simulink model "Spange_Thrust_simulation"  (R2016a)
settings: Solver=ode3  StartTime=0.0  StopTime=4  RelTol=1e-3
values from neighbouring files (symbols this model uses):
  C = [C1;C2;C3]    [Spange_init.m]
  D = 3.0/100    (= 0.03)    [Spange_init.m]
  eps_c = 5    [Spange_init.m]
  epsilon = 0.5    [Spange_init.m]
  hd = c2d(H1,0.1,'foh')    [Spange_init.m]
  hd2 = c2d(H2,0.01,'zoh')    [Spange_init.m]
  I_s = 0.05    [Spange_init.m]
  k_cc = 1    [Spange_init.m]
  K_omega = 0.3    [Spange_init.m]
  K_q1f = 0.0113    [Spange_init.m]
  K_q1r = K_q1f    (= 0.0113)    [Spange_init.m]
  K_q2f = 0.0117    [Spange_init.m]
  K_q2r = K_q2f    (= 0.0117)    [Spange_init.m]
  K_q3f = 0.0113    [Spange_init.m]
  K_q3r = K_q3f    (= 0.0113)    [Spange_init.m]
  K_T1f = 0.3763    [Spange_init.m]
  K_T1r = K_T1f    (= 0.3763)    [Spange_init.m]
  K_T2f = 0.3901    [Spange_init.m]
  K_T2r = K_T2f    (= 0.3901)    [Spange_init.m]
  K_T3f = 0.3776    [Spange_init.m]
  K_T3r = K_T3f    (= 0.3776)    [Spange_init.m]
  Kp = 0.3    [Spange_init.m]
  Max_Acceleration = 2    [Spange_init.m]
  Max_rotation = 12*sqrt(lambda)    [Spange_init.m]
  Max_thrust = 1.5034    [Spange_init.m]
  Min_thrust = -0.85    [Spange_init.m]
  n_c = 5    [Spange_init.m]
  n_max = 64.6    [Spange_init.m]
  p_cc = 0.5    [Spange_init.m]
  Q_f0 = 0.3    [Spange_init.m]
  r_cc = 4    [Spange_init.m]
  Rho = Rho_m    (= 1000)    [Spange_init.m]
  tc = [u(1),u(2),u(3)]'    [Spange_thrustallocationQuadratic_mode1.m]    (also in Spange_thrustallocationQuadratic_mode2.m; Spange_thrustallocationQuadratic_mode3.m; Spange_thrustallocationQuadratic_mode4.m)
  Thruster_control = 1    [Spange_init.m]
  u_e = [1 0 1 0 0 ... (first row only)    [Spange_init.m]
undefined symbols (not defined in the file or in its folder): Thruster
libraries: simulink_extras x4, simulink x3
settings Model: Creator=Joachim  LastModifiedBy=Joachim
settings DataIOCC: LimitDataPoints=on

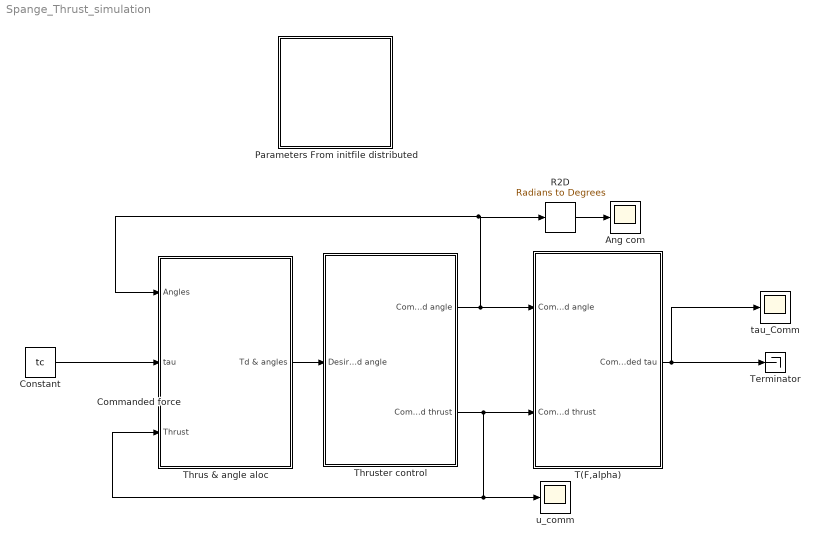
== system Spange_Thrust_simulation ==
  Ang com : Scope
  Commanded force : Constant  Value=tc
  Constant : Constant  Value=tc
  "Parameters From initfile distributed " : Subsystem
  R2D : simulink_extras/Transformations/Radians to Degrees
  T(F,alpha) : Subsystem
  Terminator : Terminator
  Thrus & angle aloc : Subsystem
  Thruster control : Subsystem
  tau_Comm : Scope
  u_comm : Scope
  wires:
  Thrus & angle aloc/1(Td & angles) -> Thruster control/1("Desired thrust and angle ")
  T(F,alpha)/1(Commanded tau) -> Terminator/1, tau_Comm/1
  R2D/1 -> Ang com/1
  Thruster control/2("Commanded thrust ") -> u_comm/1, Thrus & angle aloc/3(Thrust), T(F,alpha)/2(Commanded thrust)
  Thruster control/1(Commanded angle) -> T(F,alpha)/1(Commanded angle), R2D/1, Thrus & angle aloc/1(Angles)
  Constant/1 -> Thrus & angle aloc/2(tau)

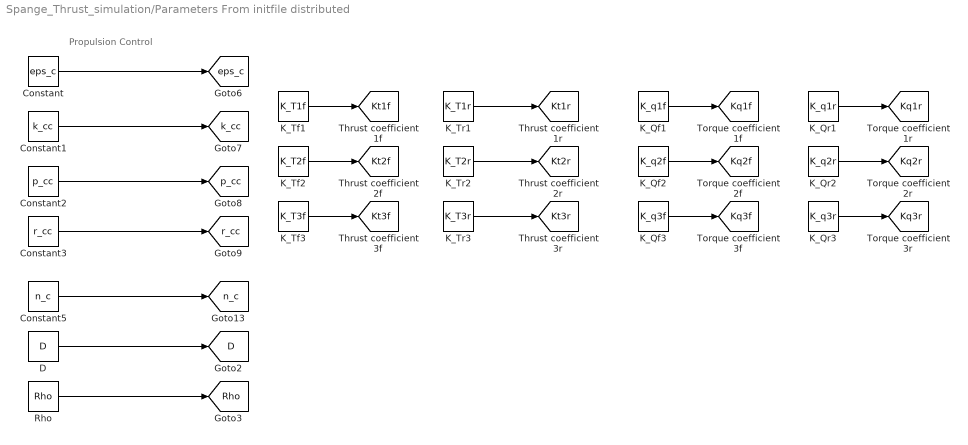
== system Spange_Thrust_simulation/Parameters From initfile distributed  ==
  note: Propulsion Control
  Constant : Constant  Value=eps_c
  Constant1 : Constant  Value=k_cc
  Constant2 : Constant  Value=p_cc
  Constant3 : Constant  Value=r_cc
  Constant5 : Constant  Value=n_c
  D : Constant  Value=D
  K_Qf1 : Constant  Value=K_q1f
  K_Qf2 : Constant  Value=K_q2f
  K_Qf3 : Constant  Value=K_q3f
  K_Qr1 : Constant  Value=K_q1r
  K_Qr2 : Constant  Value=K_q2r
  K_Qr3 : Constant  Value=K_q3r
  K_Tf1 : Constant  Value=K_T1f
  K_Tf2 : Constant  Value=K_T2f
  K_Tf3 : Constant  Value=K_T3f
  K_Tr1 : Constant  Value=K_T1r
  K_Tr2 : Constant  Value=K_T2r
  K_Tr3 : Constant  Value=K_T3r
  Rho : Constant  Value=Rho
  tag scope: D=global, Kq1f=global, Kq1r=global, Kq2f=global, Kq2r=global, Kq3f=global, Kq3r=global, Kt1f=global, Kt1r=global, Kt2f=global, Kt2r=global, Kt3f=global, Kt3r=global, Rho=global, eps_c=global, k_cc=global, n_c=global, p_cc=global, r_cc=global
  wires:
  D/1 -> [D]
  Rho/1 -> [Rho]
  Constant/1 -> [eps_c]
  Constant1/1 -> [k_cc]
  Constant2/1 -> [p_cc]
  Constant3/1 -> [r_cc]
  Constant5/1 -> [n_c]
  K_Tf1/1 -> [Kt1f]
  K_Tf3/1 -> [Kt3f]
  K_Tf2/1 -> [Kt2f]
  K_Tr1/1 -> [Kt1r]
  K_Tr2/1 -> [Kt2r]
  K_Tr3/1 -> [Kt3r]
  K_Qf1/1 -> [Kq1f]
  K_Qf2/1 -> [Kq2f]
  K_Qf3/1 -> [Kq3f]
  K_Qr1/1 -> [Kq1r]
  K_Qr2/1 -> [Kq2r]
  K_Qr3/1 -> [Kq3r]

== system Spange_Thrust_simulation/T(F,alpha) ==
  Commanded angle : Inport
  Commanded thrust : Inport  Port=2
  MATLAB Function : MATLAB Function  TreatAsAtomicUnit=on
  Radians to Degrees : simulink_extras/Transformations/Radians to Degrees
  X-position Thruster : Constant  Value=[Thruster.T1(1) Thruster.T2(1) Thruster.T3(1)]
  Y-position Thruster : Constant  Value=[Thruster.T1(2) Thruster.T2(2) Thruster.T3(2)]
  Commanded tau : Outport
  wires:
  Commanded angle/1 -> Radians to Degrees/1
  X-position Thruster/1 -> MATLAB Function/3(PosX)
  Y-position Thruster/1 -> MATLAB Function/4(PosY)
  MATLAB Function/1(actual_tau) -> Commanded tau/1
  Commanded thrust/1 -> MATLAB Function/1(thrust_actual)
  Radians to Degrees/1 -> MATLAB Function/2(alpha_actual)

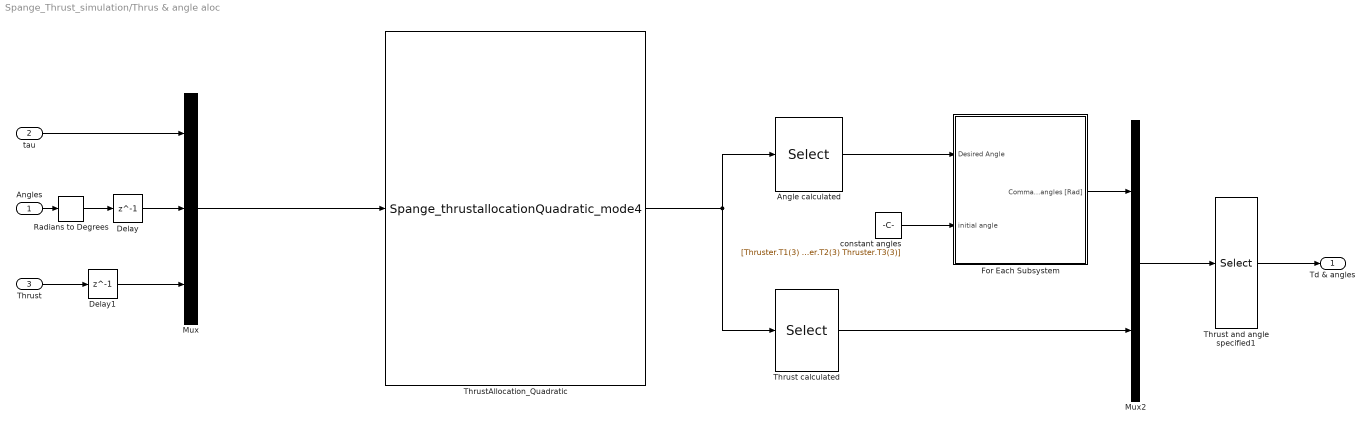
== system Spange_Thrust_simulation/Thrus & angle aloc ==
  Angles : Inport
  tau : Inport  Port=2
  Thrust : Inport  Port=3
  "  Thrust calculated" : Selector  InputPortWidth=6  IndexOptions=Index vector (dialog)  Indices=[4 5 6]  OutputSizes=1
  " Angle calculated" : Selector  InputPortWidth=6  IndexOptions=Index vector (dialog)  Indices=[1 2 3]  OutputSizes=1
  Delay : Delay  DelayLength=1  InitialCondition=[Thruster.T1(3) Thruster.T2(3) Thruster.T3(3)]
  Delay1 : Delay  DelayLength=1  InitialCondition=[0,0,0]
  For Each Subsystem : Subsystem  TreatAsAtomicUnit=on
  Mux : Mux  Inputs=3
  Mux2 : Mux  Inputs=2
  Radians to Degrees : simulink_extras/Transformations/Radians to Degrees
  Thrust and angle specified1 : Selector  InputPortWidth=6  IndexOptions=Index vector (dialog)  Indices=[4 1 5 2 6 3]  OutputSizes=1
  ThrustAllocation_Quadratic : S-Function  RequirementInfo={} %GIDa_b9c7dd03_57d1_40a3_b341_131bae047cf5  FunctionName=Spange_thrustallocationQuadratic_mode4  Parameters=u_e,Thruster,C  SFunctionDeploymentMode=off  EnableBusSupport=off
  constant angles : Constant  Value=[Thruster.T1(3) Thruster.T2(3) Thruster.T3(3)]
  Td & angles : Outport
  wires:
  tau/1 -> Mux/1
  Angles/1 -> Radians to Degrees/1
  Radians to Degrees/1 -> Delay/1
  Thrust/1 -> Delay1/1
  Delay/1 -> Mux/2
  Thrust and angle specified1/1 -> Td & angles/1
  Mux2/1 -> Thrust and angle specified1/1
  " Angle calculated"/1 -> For Each Subsystem/1(Desired Angle)
  For Each Subsystem/1("Commanded angles [Rad] ") -> Mux2/1
  constant angles/1 -> For Each Subsystem/2("initial angle ")
  "  Thrust calculated"/1 -> Mux2/2
  ThrustAllocation_Quadratic/1 -> " Angle calculated"/1, "  Thrust calculated"/1
  Delay1/1 -> Mux/3
  Mux/1 -> ThrustAllocation_Quadratic/1

== system Spange_Thrust_simulation/Thruster control ==
  "Desired thrust and angle " : Inport
  Demux : Demux  Outputs=6
  Mux : Mux  Inputs=6
  Selecting Actual thrust : Selector  InputPortWidth=6  IndexOptions=Index vector (dialog)  Indices=[1 3 5]  OutputSizes=1
  Selecting actual angle : Selector  InputPortWidth=6  IndexOptions=Index vector (dialog)  Indices=[2 4 6]  OutputSizes=1
  Subsystem : Subsystem
  Thruster 1 : Subsystem
      settings: AttributesFormatString=%<MinAlgLoopOccurrences>
  Thruster 2 : Subsystem
      settings: AttributesFormatString=%<MinAlgLoopOccurrences>
  Thruster 3 : Subsystem
      settings: AttributesFormatString=%<MinAlgLoopOccurrences>
  Commanded angle : Outport
  "Commanded thrust " : Outport  Port=2
  wires:
  Demux/1 -> Thruster 1/1(Desired thrust 1)
  Selecting Actual thrust/1 -> Subsystem/1(Calculated thrust)
  Subsystem/1(Thrust from model) -> "Commanded thrust "/1
  Selecting actual angle/1 -> Commanded angle/1
  Thruster 1/2(Commanded angle) -> Mux/2
  Demux/2 -> Thruster 1/2(Desired Angle)
  Mux/1 -> Selecting Actual thrust/1, Selecting actual angle/1
  Thruster 3/2(Commanded angle) -> Mux/6
  Thruster 3/1("Commanded thrust ") -> Mux/5
  Thruster 2/2(Commanded angle) -> Mux/4
  Thruster 2/1(Commanded thrust 1) -> Mux/3
  Thruster 1/1(Commanded thrust 1) -> Mux/1
  Demux/6 -> Thruster 3/2(Desired Angle)
  Demux/5 -> Thruster 3/1(Desired thrust 1)
  Demux/4 -> Thruster 2/2(Desired Angle)
  Demux/3 -> Thruster 2/1(Desired thrust 1)
  "Desired thrust and angle "/1 -> Demux/1

== system Spange_Thrust_simulation/Thrus & angle aloc/For Each Subsystem ==
  Desired Angle : Inport  Partition=on  PartitionDimension=1  PartitionWidth=1
  "initial angle " : Inport  Port=2  Partition=on  PartitionDimension=1  PartitionWidth=1
  Degrees to Radians : simulink_extras/Transformations/Degrees to Radians
  Ensures fastest way is chosen : MATLAB Function  TreatAsAtomicUnit=on
  For Each : ForEach  DisableCoverage=on  IndexMode=One-based
  Integrator : Integrator  ExternalReset=either  InitialConditionSource=external
  MATLAB Function : MATLAB Function  TreatAsAtomicUnit=on
  Max Rotation Rate : Saturate  UpperLimit=Max_rotation  LowerLimit=-Max_rotation
  constant : Constant  Value=0
  "Commanded angles [Rad] " : Outport  ConcatenationDimension=1
  wires:
  Degrees to Radians/1 -> MATLAB Function/1(angle)
  MATLAB Function/1(y) -> "Commanded angles [Rad] "/1
  Integrator/1 -> Degrees to Radians/1, Ensures fastest way is chosen/2(actual)  "angle"
  "initial angle "/1 -> Integrator/3
  Max Rotation Rate/1 -> Integrator/1
  Ensures fastest way is chosen/1(psi_D) -> Max Rotation Rate/1
  Desired Angle/1 -> Ensures fastest way is chosen/1(desired)
  constant/1 -> Integrator/2

== system Spange_Thrust_simulation/Thruster control/Subsystem ==
  Calculated thrust : Inport
  Demux : Demux  Outputs=3
  Mux : Mux  Inputs=3
  Saturation 1 : Saturate  UpperLimit=Max_thrust  LowerLimit=Min_thrust
  Saturation 2 : Saturate  UpperLimit=Max_thrust  LowerLimit=Min_thrust
  Saturation 3 : Saturate  UpperLimit=Max_thrust  LowerLimit=Min_thrust
  Thrust from model : Outport
  wires:
  Saturation 2/1 -> Mux/2
  Saturation 3/1 -> Mux/3
  Saturation 1/1 -> Mux/1
  Mux/1 -> Thrust from model/1
  Demux/3 -> Saturation 3/1
  Demux/2 -> Saturation 2/1
  Demux/1 -> Saturation 1/1
  Calculated thrust/1 -> Demux/1

== system Spange_Thrust_simulation/Thruster control/Thruster 1 ==
  Desired thrust 1 : Inport
  Desired Angle : Inport  Port=2
  Constant : Constant  Value=hd2.den{1,1}
  Constant1 : Constant  Value=hd2.num{1,1}
  Discrete Transfer Fcn : DiscreteTransferFcn  NumeratorSource=Input port  DenominatorSource=Input port  Denominator=[0.2 1]  SampleTime=0.01  a0EqualsOne=on
      settings: InputPortMap=u0,p1,p3
  Losses (placeholder) : Constant  Value=0
  Propeller Hydrodynamics : Subsystem
  Shaft dynamics : Subsystem
  Thruster control : Subsystem
  Commanded thrust 1 : Outport
  Commanded angle : Outport  Port=2
  wires:
  Desired thrust 1/1 -> Thruster control/1("T_d ")
  Discrete Transfer Fcn/1 -> Shaft dynamics/1(Qm)
  Propeller Hydrodynamics/2(Qa) -> Shaft dynamics/2(Qa)
  Shaft dynamics/1(n) -> Propeller Hydrodynamics/2(n), Thruster control/2(n)
  Constant/1 -> Discrete Transfer Fcn/3
  Constant1/1 -> Discrete Transfer Fcn/2
  Desired Angle/1 -> Commanded angle/1
  Thruster control/1(Qc) -> Discrete Transfer Fcn/1
  Propeller Hydrodynamics/1(Ta) -> Commanded thrust 1/1
  Losses (placeholder)/1 -> Propeller Hydrodynamics/1(env)

== system Spange_Thrust_simulation/Thruster control/Thruster 2 ==
  Desired thrust 1 : Inport
  Desired Angle : Inport  Port=2
  Constant : Constant  Value=hd2.den{1,1}
  Constant1 : Constant  Value=hd2.num{1,1}
  Discrete Transfer Fcn : DiscreteTransferFcn  NumeratorSource=Input port  DenominatorSource=Input port  Denominator=[0.2 1]  SampleTime=0.01  a0EqualsOne=on
      settings: InputPortMap=u0,p1,p3
  Losses (placeholder) : Constant  Value=0
  Propeller Hydrodynamics : Subsystem
  Shaft dynamics : Subsystem
  Thruster control : Subsystem
  Commanded thrust 1 : Outport
  Commanded angle : Outport  Port=2
  wires:
  Propeller Hydrodynamics/2(Qa) -> Shaft dynamics/2(Qa)
  Shaft dynamics/1(n) -> Propeller Hydrodynamics/2(n), Thruster control/2(n)
  Constant/1 -> Discrete Transfer Fcn/3
  Constant1/1 -> Discrete Transfer Fcn/2
  Desired Angle/1 -> Commanded angle/1
  Propeller Hydrodynamics/1(Ta) -> Commanded thrust 1/1
  Desired thrust 1/1 -> Thruster control/1("T_d ")
  Discrete Transfer Fcn/1 -> Shaft dynamics/1(Qm)
  Thruster control/1(Qc) -> Discrete Transfer Fcn/1
  Losses (placeholder)/1 -> Propeller Hydrodynamics/1(env)

== system Spange_Thrust_simulation/Thruster control/Thruster 3 ==
  Desired thrust 1 : Inport
  Desired Angle : Inport  Port=2
  Constant : Constant  Value=hd2.den{1,1}
  Constant1 : Constant  Value=hd2.num{1,1}
  Discrete Transfer Fcn : DiscreteTransferFcn  NumeratorSource=Input port  DenominatorSource=Input port  Denominator=[0.2 1]  SampleTime=0.01  a0EqualsOne=on
      settings: InputPortMap=u0,p1,p3
  Losses (placeholder) : Constant  Value=0
  Propeller Hydrodynamics : Subsystem
  Shaft dynamics : Subsystem
  Thruster control : Subsystem
  "Commanded thrust " : Outport
  Commanded angle : Outport  Port=2
  wires:
  Propeller Hydrodynamics/2(Qa) -> Shaft dynamics/2(Qa)
  Shaft dynamics/1(n) -> Propeller Hydrodynamics/2(n), Thruster control/2(n)
  Constant/1 -> Discrete Transfer Fcn/3
  Constant1/1 -> Discrete Transfer Fcn/2
  Desired Angle/1 -> Commanded angle/1
  Propeller Hydrodynamics/1(Ta) -> "Commanded thrust "/1
  Desired thrust 1/1 -> Thruster control/1("T_d ")
  Discrete Transfer Fcn/1 -> Shaft dynamics/1(Qm)
  Thruster control/1(Qc) -> Discrete Transfer Fcn/1
  Losses (placeholder)/1 -> Propeller Hydrodynamics/1(env)

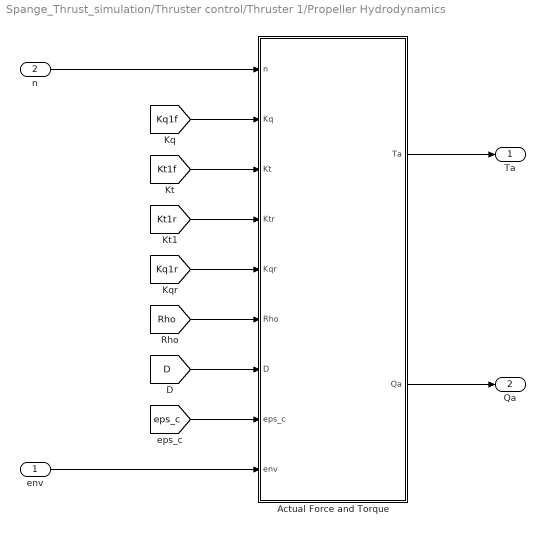
== system Spange_Thrust_simulation/Thruster control/Thruster 1/Propeller Hydrodynamics ==
  env : Inport
  n : Inport  Port=2
  Actual Force and Torque : MATLAB Function  TreatAsAtomicUnit=on
  Ta : Outport
  Qa : Outport  Port=2
  wires:
  [eps_c] -> Actual Force and Torque/8(eps_c)
  [Kq1r] -> Actual Force and Torque/5(Kqr)
  [Kt1r] -> Actual Force and Torque/4(Ktr)
  Actual Force and Torque/1(Ta) -> Ta/1
  [Kt1f] -> Actual Force and Torque/3(Kt)
  env/1 -> Actual Force and Torque/9(env)
  [Rho] -> Actual Force and Torque/6(Rho)
  Actual Force and Torque/2(Qa) -> Qa/1
  [Kq1f] -> Actual Force and Torque/2(Kq)
  [D] -> Actual Force and Torque/7(D)
  n/1 -> Actual Force and Torque/1(n)

== system Spange_Thrust_simulation/Thruster control/Thruster 1/Shaft dynamics ==
  Qm : Inport
  Qa : Inport  Port=2
  Constant : Constant  Value=0
  Finding rotation speed : Gain  Gain=1/(2*pi*I_s)
  Integrator : Integrator  ExternalReset=either
  K_omega : Gain  Gain=K_omega*2*pi
  Sum : Sum  Inputs=-+-
  n : Outport
  wires:
  Constant/1 -> Integrator/2
  Integrator/1 -> K_omega/1, n/1
  Finding rotation speed/1 -> Integrator/1
  K_omega/1 -> Sum/3
  Qa/1 -> Sum/1
  Sum/1 -> Finding rotation speed/1
  Qm/1 -> Sum/2

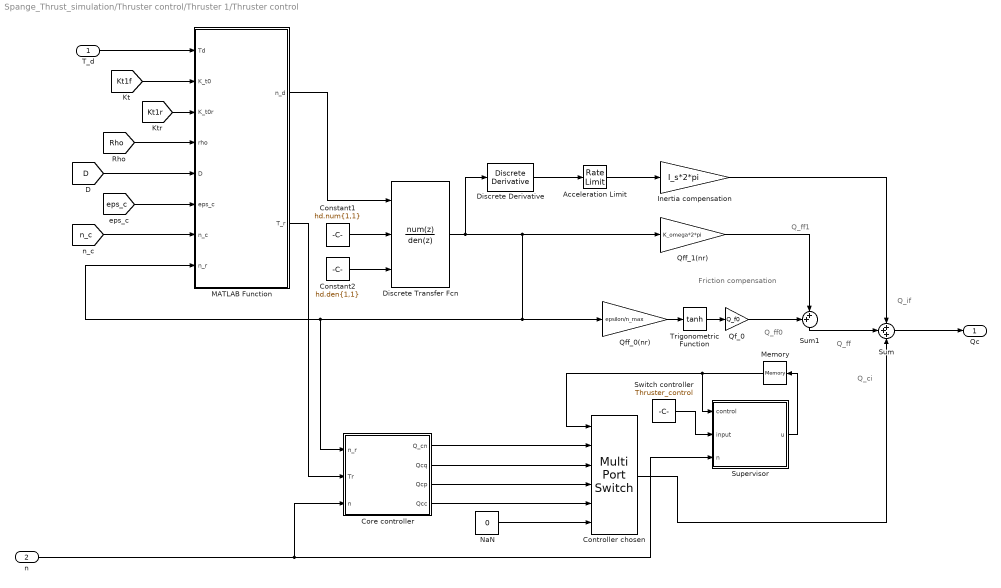
== system Spange_Thrust_simulation/Thruster control/Thruster 1/Thruster control ==
  note: Friction compensation
  note: Q_ff1
  note: Q_ff0
  note: Q_ff
  note: Q_if
  note: Q_ci
  "T_d " : Inport
  n : Inport  Port=2
  Acceleration Limit : RateLimiter  RisingSlewLimit=Max_Acceleration  FallingSlewLimit=-Max_Acceleration  SampleTimeMode=inherited
  Constant1 : Constant  Value=hd.num{1,1}  VectorParams1D=off
  Constant2 : Constant  Value=hd.den{1,1}  VectorParams1D=off
  Controller chosen : MultiPortSwitch  Inputs=5
  Core controller : Subsystem
  Discrete Transfer Fcn : DiscreteTransferFcn  NumeratorSource=Input port  Numerator=[8.76e-05 0.0003481 8.648e-05]  DenominatorSource=Input port  Denominator=[1 -1.974 0.9746]  SampleTime=0.01  a0EqualsOne=on
      settings: InputPortMap=u0,p1,p3
  Discrete Derivative : simulink/Discrete/Discrete Derivative  gainval=1.0  ICPrevScaledInput=0.0  InputProcessing=Inherited  OutMin=[]  OutMax=[]  OutDataType=fixdt(1, 16)  OutScaling=2^-10  DoSatur=off
  Inertia compensation : Gain  Gain=I_s*2*pi
  MATLAB Function : MATLAB Function  TreatAsAtomicUnit=on
  Memory : Memory  X0=1  InheritSampleTime=on
  NaN : Constant  Value=0
  Qf_0 : Gain  Gain=Q_f0
  Qff_0(nr) : Gain  Gain=epsilon/n_max
  Qff_1(nr) : Gain  Gain=K_omega*2*pi
  Sum : Sum  Inputs=+++
  Sum1 : Sum  Inputs=++|
  Supervisor : MATLAB Function  TreatAsAtomicUnit=on
  Switch controller : Constant  Value=Thruster_control
  Trigonometric Function : Trigonometry  Operator=tanh
  Qc : Outport
  wires:
  Sum/1 -> Qc/1
  [Kt1r] -> MATLAB Function/3(K_t0r)
  [Kt1f] -> MATLAB Function/2(K_t0)
  "T_d "/1 -> MATLAB Function/1(Td)
  Discrete Transfer Fcn/1 -> Discrete Derivative/1, Qff_1(nr)/1, Qff_0(nr)/1, MATLAB Function/8(n_r), Core controller/1(n_r)
  Acceleration Limit/1 -> Inertia compensation/1
  n/1 -> Supervisor/3(n), Core controller/3("n ")
  Inertia compensation/1 -> Sum/1
  Constant2/1 -> Discrete Transfer Fcn/3
  Constant1/1 -> Discrete Transfer Fcn/2
  Sum1/1 -> Sum/2
  Discrete Derivative/1 -> Acceleration Limit/1
  [n_c] -> MATLAB Function/7(n_c)
  Core controller/1(Q_cn) -> Controller chosen/2
  Core controller/4(Qcc) -> Controller chosen/5
  Core controller/3(Qcp) -> Controller chosen/4
  Core controller/2(Qcq) -> Controller chosen/3
  Controller chosen/1 -> Sum/3
  Switch controller/1 -> Supervisor/2(input)
  Qf_0/1 -> Sum1/1
  Qff_1(nr)/1 -> Sum1/2
  Memory/1 -> Supervisor/1(control), Controller chosen/1
  Supervisor/1(u) -> Memory/1
  NaN/1 -> Controller chosen/6
  Trigonometric Function/1 -> Qf_0/1
  Qff_0(nr)/1 -> Trigonometric Function/1
  MATLAB Function/1(n_d) -> Discrete Transfer Fcn/1
  MATLAB Function/2(T_r) -> Core controller/2("Tr ")
  [eps_c] -> MATLAB Function/6(eps_c)
  [D] -> MATLAB Function/5(D)
  [Rho] -> MATLAB Function/4(rho)

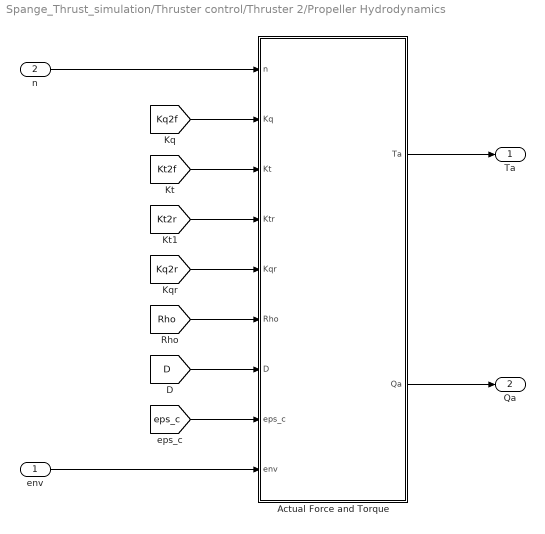
== system Spange_Thrust_simulation/Thruster control/Thruster 2/Propeller Hydrodynamics ==
  env : Inport
  n : Inport  Port=2
  Actual Force and Torque : MATLAB Function  TreatAsAtomicUnit=on
  Ta : Outport
  Qa : Outport  Port=2
  wires:
  [eps_c] -> Actual Force and Torque/8(eps_c)
  [Kq2r] -> Actual Force and Torque/5(Kqr)
  [Kt2r] -> Actual Force and Torque/4(Ktr)
  Actual Force and Torque/1(Ta) -> Ta/1
  [Kt2f] -> Actual Force and Torque/3(Kt)
  env/1 -> Actual Force and Torque/9(env)
  [Rho] -> Actual Force and Torque/6(Rho)
  Actual Force and Torque/2(Qa) -> Qa/1
  [Kq2f] -> Actual Force and Torque/2(Kq)
  [D] -> Actual Force and Torque/7(D)
  n/1 -> Actual Force and Torque/1(n)

== system Spange_Thrust_simulation/Thruster control/Thruster 2/Shaft dynamics ==
  Qm : Inport
  Qa : Inport  Port=2
  Constant : Constant  Value=0
  Finding rotation speed : Gain  Gain=1/(2*pi*I_s)
  Integrator : Integrator  ExternalReset=either
  K_omega : Gain  Gain=K_omega*2*pi
  Sum : Sum  Inputs=-+-
  n : Outport
  wires:
  Constant/1 -> Integrator/2
  Integrator/1 -> n/1, K_omega/1
  Finding rotation speed/1 -> Integrator/1
  K_omega/1 -> Sum/3
  Qa/1 -> Sum/1
  Sum/1 -> Finding rotation speed/1
  Qm/1 -> Sum/2

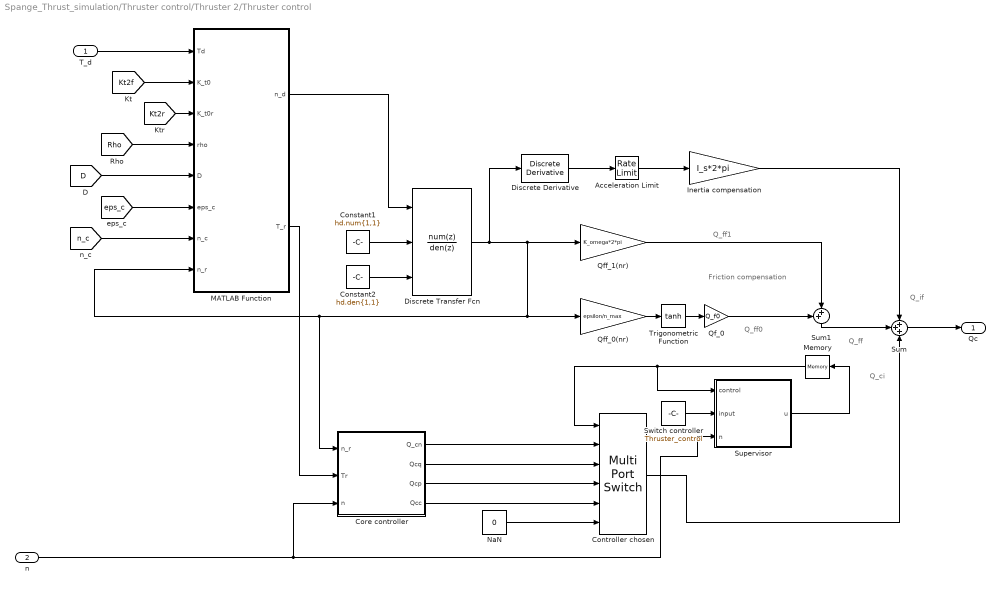
== system Spange_Thrust_simulation/Thruster control/Thruster 2/Thruster control ==
  note: Friction compensation
  note: Q_ff1
  note: Q_ff0
  note: Q_ff
  note: Q_if
  note: Q_ci
  "T_d " : Inport
  n : Inport  Port=2
  Acceleration Limit : RateLimiter  RisingSlewLimit=Max_Acceleration  FallingSlewLimit=-Max_Acceleration  SampleTimeMode=inherited
  Constant1 : Constant  Value=hd.num{1,1}  VectorParams1D=off
  Constant2 : Constant  Value=hd.den{1,1}  VectorParams1D=off
  Controller chosen : MultiPortSwitch  Inputs=5
  Core controller : Subsystem
  Discrete Transfer Fcn : DiscreteTransferFcn  NumeratorSource=Input port  Numerator=[8.76e-05 0.0003481 8.648e-05]  DenominatorSource=Input port  Denominator=[1 -1.974 0.9746]  SampleTime=0.01  a0EqualsOne=on
      settings: InputPortMap=u0,p1,p3
  Discrete Derivative : simulink/Discrete/Discrete Derivative  gainval=1.0  ICPrevScaledInput=0.0  InputProcessing=Inherited  OutMin=[]  OutMax=[]  OutDataType=fixdt(1, 16)  OutScaling=2^-10  DoSatur=off
  Inertia compensation : Gain  Gain=I_s*2*pi
  MATLAB Function : MATLAB Function  TreatAsAtomicUnit=on
  Memory : Memory  X0=1
  NaN : Constant  Value=0
  Qf_0 : Gain  Gain=Q_f0
  Qff_0(nr) : Gain  Gain=epsilon/n_max
  Qff_1(nr) : Gain  Gain=K_omega*2*pi
  Sum : Sum  Inputs=+++
  Sum1 : Sum  Inputs=++|
  Supervisor : MATLAB Function  TreatAsAtomicUnit=on
  Switch controller : Constant  Value=Thruster_control
  Trigonometric Function : Trigonometry  Operator=tanh
  Qc : Outport
  wires:
  [Kt2r] -> MATLAB Function/3(K_t0r)
  [Kt2f] -> MATLAB Function/2(K_t0)
  Sum/1 -> Qc/1
  Discrete Transfer Fcn/1 -> Qff_1(nr)/1, Core controller/1(n_r), MATLAB Function/8(n_r), Qff_0(nr)/1, Discrete Derivative/1
  Acceleration Limit/1 -> Inertia compensation/1
  n/1 -> Supervisor/3(n), Core controller/3("n ")
  Discrete Derivative/1 -> Acceleration Limit/1
  MATLAB Function/1(n_d) -> Discrete Transfer Fcn/1
  Constant2/1 -> Discrete Transfer Fcn/3
  Constant1/1 -> Discrete Transfer Fcn/2
  [n_c] -> MATLAB Function/7(n_c)
  [eps_c] -> MATLAB Function/6(eps_c)
  [D] -> MATLAB Function/5(D)
  [Rho] -> MATLAB Function/4(rho)
  "T_d "/1 -> MATLAB Function/1(Td)
  Switch controller/1 -> Supervisor/2(input)
  Core controller/2(Qcq) -> Controller chosen/3
  Core controller/3(Qcp) -> Controller chosen/4
  Inertia compensation/1 -> Sum/1
  Controller chosen/1 -> Sum/3
  Qf_0/1 -> Sum1/1
  Qff_1(nr)/1 -> Sum1/2
  Memory/1 -> Controller chosen/1, Supervisor/1(control)
  Supervisor/1(u) -> Memory/1
  NaN/1 -> Controller chosen/6
  Core controller/4(Qcc) -> Controller chosen/5
  Core controller/1(Q_cn) -> Controller chosen/2
  Sum1/1 -> Sum/2
  Trigonometric Function/1 -> Qf_0/1
  Qff_0(nr)/1 -> Trigonometric Function/1
  MATLAB Function/2(T_r) -> Core controller/2("Tr ")

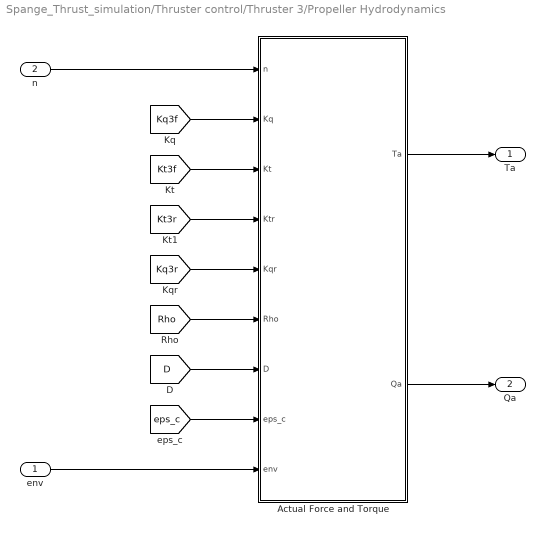
== system Spange_Thrust_simulation/Thruster control/Thruster 3/Propeller Hydrodynamics ==
  env : Inport
  n : Inport  Port=2
  Actual Force and Torque : MATLAB Function  TreatAsAtomicUnit=on
  Ta : Outport
  Qa : Outport  Port=2
  wires:
  [eps_c] -> Actual Force and Torque/8(eps_c)
  [Kq3r] -> Actual Force and Torque/5(Kqr)
  [Kt3r] -> Actual Force and Torque/4(Ktr)
  Actual Force and Torque/1(Ta) -> Ta/1
  [Kt3f] -> Actual Force and Torque/3(Kt)
  env/1 -> Actual Force and Torque/9(env)
  [Rho] -> Actual Force and Torque/6(Rho)
  Actual Force and Torque/2(Qa) -> Qa/1
  [Kq3f] -> Actual Force and Torque/2(Kq)
  [D] -> Actual Force and Torque/7(D)
  n/1 -> Actual Force and Torque/1(n)

== system Spange_Thrust_simulation/Thruster control/Thruster 3/Shaft dynamics ==
  Qm : Inport
  Qa : Inport  Port=2
  Constant : Constant  Value=0
  Finding rotation speed : Gain  Gain=1/(2*pi*I_s)
  Integrator : Integrator  ExternalReset=either
  K_omega : Gain  Gain=K_omega*2*pi
  Sum : Sum  Inputs=-+-
  n : Outport
  wires:
  Constant/1 -> Integrator/2
  Integrator/1 -> K_omega/1, n/1
  Finding rotation speed/1 -> Integrator/1
  K_omega/1 -> Sum/3
  Qa/1 -> Sum/1
  Sum/1 -> Finding rotation speed/1
  Qm/1 -> Sum/2

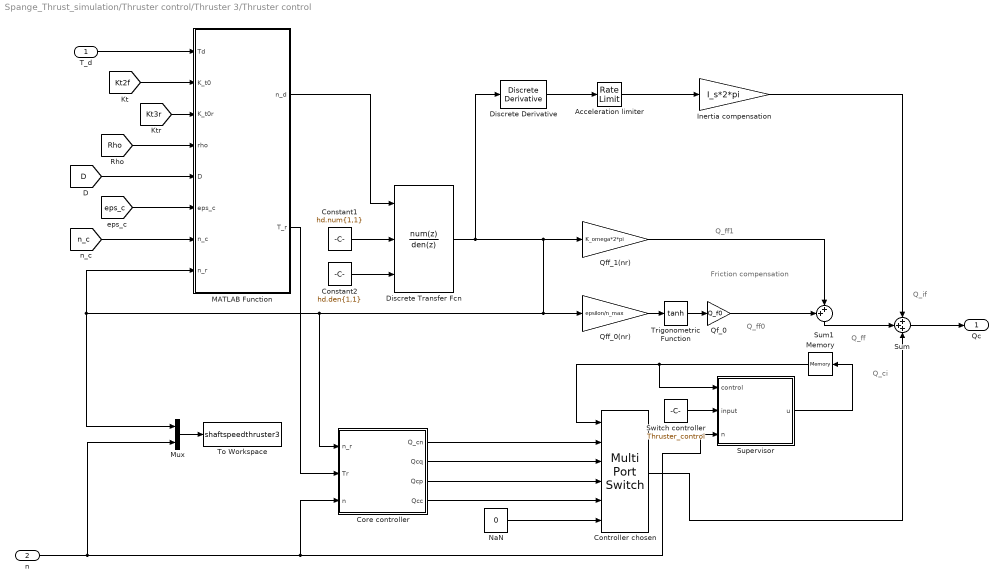
== system Spange_Thrust_simulation/Thruster control/Thruster 3/Thruster control ==
  note: Friction compensation
  note: Q_ff1
  note: Q_ff0
  note: Q_ff
  note: Q_if
  note: Q_ci
  "T_d " : Inport
  n : Inport  Port=2
  Acceleration limiter : RateLimiter  RisingSlewLimit=Max_Acceleration  FallingSlewLimit=-Max_Acceleration  SampleTimeMode=inherited
  Constant1 : Constant  Value=hd.num{1,1}  VectorParams1D=off
  Constant2 : Constant  Value=hd.den{1,1}  VectorParams1D=off
  Controller chosen : MultiPortSwitch  Inputs=5
  Core controller : Subsystem
  Discrete Transfer Fcn : DiscreteTransferFcn  NumeratorSource=Input port  Numerator=[8.76e-05 0.0003481 8.648e-05]  DenominatorSource=Input port  Denominator=[1 -1.974 0.9746]  SampleTime=0.01  a0EqualsOne=on
      settings: InputPortMap=u0,p1,p3
  Discrete Derivative : simulink/Discrete/Discrete Derivative  gainval=1.0  ICPrevScaledInput=0.0  InputProcessing=Inherited  OutMin=[]  OutMax=[]  OutDataType=fixdt(1, 16)  OutScaling=2^-10  DoSatur=off
  Inertia compensation : Gain  Gain=I_s*2*pi
  MATLAB Function : MATLAB Function  TreatAsAtomicUnit=on
  Memory : Memory  X0=1
  Mux : Mux  Inputs=2
  NaN : Constant  Value=0
  Qf_0 : Gain  Gain=Q_f0
  Qff_0(nr) : Gain  Gain=epsilon/n_max
  Qff_1(nr) : Gain  Gain=K_omega*2*pi
  Sum : Sum  Inputs=+++
  Sum1 : Sum  Inputs=++|
  Supervisor : MATLAB Function  TreatAsAtomicUnit=on
  Switch controller : Constant  Value=Thruster_control
  To Workspace : ToWorkspace  VariableName=shaftspeedthruster3  SaveFormat=Timeseries  SampleTime=-1
  Trigonometric Function : Trigonometry  Operator=tanh
  Qc : Outport
  wires:
  [Kt3r] -> MATLAB Function/3(K_t0r)
  [Kt2f] -> MATLAB Function/2(K_t0)
  Sum/1 -> Qc/1
  Discrete Transfer Fcn/1 -> Qff_1(nr)/1, Qff_0(nr)/1, Core controller/1(n_r), Mux/1, MATLAB Function/8(n_r), Discrete Derivative/1
  Acceleration limiter/1 -> Inertia compensation/1
  Mux/1 -> To Workspace/1
  n/1 -> Supervisor/3(n), Core controller/3("n "), Mux/2
  MATLAB Function/1(n_d) -> Discrete Transfer Fcn/1
  Constant2/1 -> Discrete Transfer Fcn/3
  Constant1/1 -> Discrete Transfer Fcn/2
  [n_c] -> MATLAB Function/7(n_c)
  [eps_c] -> MATLAB Function/6(eps_c)
  [D] -> MATLAB Function/5(D)
  [Rho] -> MATLAB Function/4(rho)
  "T_d "/1 -> MATLAB Function/1(Td)
  Switch controller/1 -> Supervisor/2(input)
  Core controller/2(Qcq) -> Controller chosen/3
  Core controller/3(Qcp) -> Controller chosen/4
  Inertia compensation/1 -> Sum/1
  Controller chosen/1 -> Sum/3
  Qf_0/1 -> Sum1/1
  Qff_1(nr)/1 -> Sum1/2
  Memory/1 -> Controller chosen/1, Supervisor/1(control)
  Supervisor/1(u) -> Memory/1
  NaN/1 -> Controller chosen/6
  Core controller/4(Qcc) -> Controller chosen/5
  Core controller/1(Q_cn) -> Controller chosen/2
  Sum1/1 -> Sum/2
  Trigonometric Function/1 -> Qf_0/1
  Qff_0(nr)/1 -> Trigonometric Function/1
  Discrete Derivative/1 -> Acceleration limiter/1
  MATLAB Function/2(T_r) -> Core controller/2("Tr ")

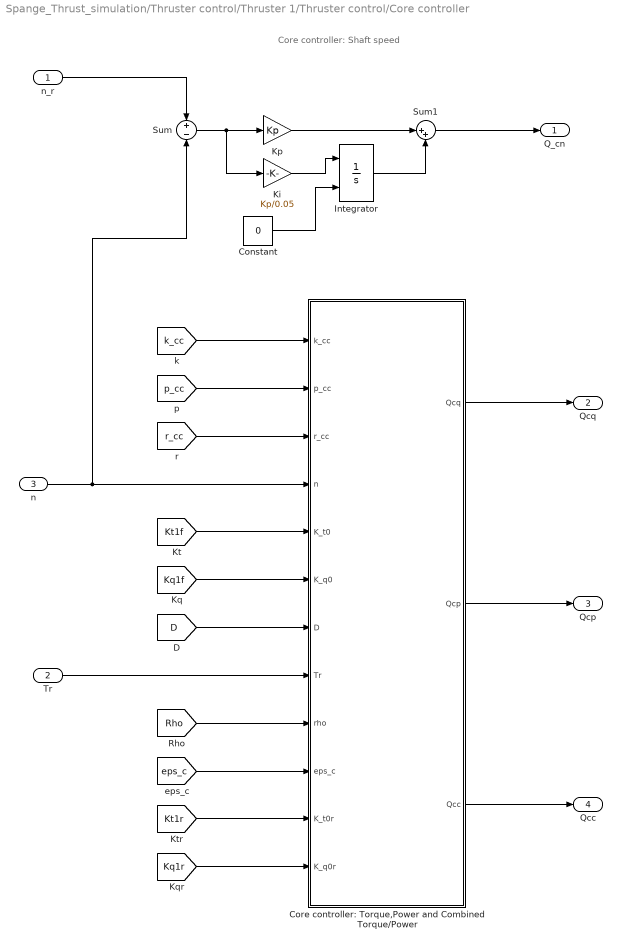
== system Spange_Thrust_simulation/Thruster control/Thruster 1/Thruster control/Core controller ==
  note: Core controller: Shaft speed
  n_r : Inport
  "Tr " : Inport  Port=2
  "n " : Inport  Port=3
  Constant : Constant  Value=0
  Core controller: Torque,Power and Combined Torque/Power : MATLAB Function  TreatAsAtomicUnit=on
  Integrator : Integrator  ExternalReset=either
  Ki : Gain  Gain=Kp/0.05
  Kp : Gain  Gain=Kp
  Sum : Sum  Inputs=+|-
  Sum1 : Sum  Inputs=|++
  Q_cn : Outport
  Qcq : Outport  Port=2
  Qcp : Outport  Port=3
  Qcc : Outport  Port=4
  wires:
  [Kq1r] -> Core controller: Torque,Power and Combined Torque/Power/12(K_q0r)
  [Kq1f] -> Core controller: Torque,Power and Combined Torque/Power/6(K_q0)
  [Kt1r] -> Core controller: Torque,Power and Combined Torque/Power/11(K_t0r)
  [eps_c] -> Core controller: Torque,Power and Combined Torque/Power/10(eps_c)
  Constant/1 -> Integrator/2
  Sum/1 -> Kp/1, Ki/1
  Sum1/1 -> Q_cn/1
  Integrator/1 -> Sum1/2
  Kp/1 -> Sum1/1
  Ki/1 -> Integrator/1
  n_r/1 -> Sum/1
  Core controller: Torque,Power and Combined Torque/Power/1(Qcq) -> Qcq/1
  Core controller: Torque,Power and Combined Torque/Power/2(Qcp) -> Qcp/1
  "Tr "/1 -> Core controller: Torque,Power and Combined Torque/Power/8(Tr)
  "n "/1 -> Core controller: Torque,Power and Combined Torque/Power/4(n), Sum/2
  [Rho] -> Core controller: Torque,Power and Combined Torque/Power/9(rho)
  [D] -> Core controller: Torque,Power and Combined Torque/Power/7(D)
  [Kt1f] -> Core controller: Torque,Power and Combined Torque/Power/5(K_t0)
  Core controller: Torque,Power and Combined Torque/Power/3(Qcc) -> Qcc/1
  [r_cc] -> Core controller: Torque,Power and Combined Torque/Power/3(r_cc)
  [p_cc] -> Core controller: Torque,Power and Combined Torque/Power/2(p_cc)
  [k_cc] -> Core controller: Torque,Power and Combined Torque/Power/1(k_cc)

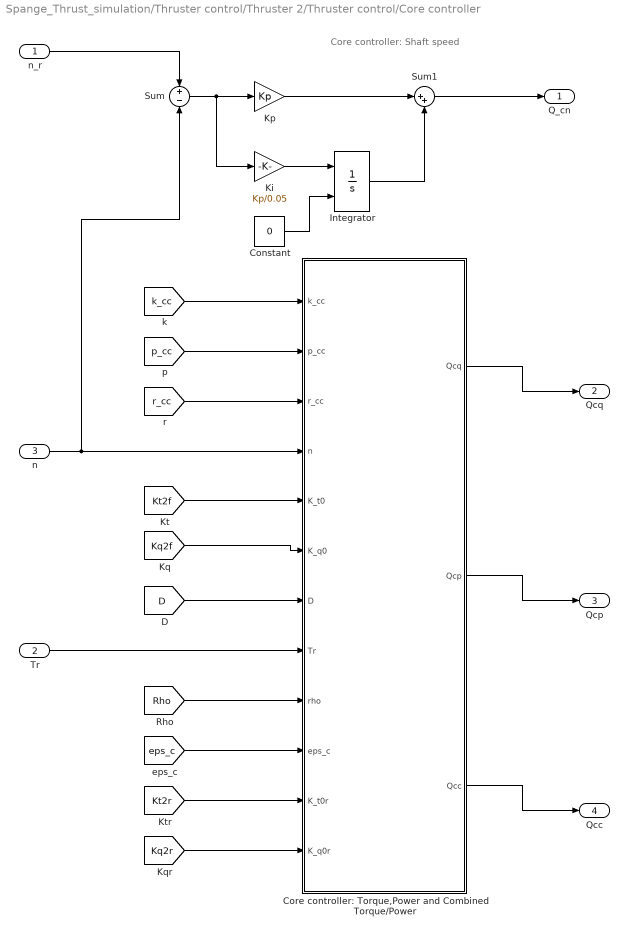
== system Spange_Thrust_simulation/Thruster control/Thruster 2/Thruster control/Core controller ==
  note: Core controller: Shaft speed
  n_r : Inport
  "Tr " : Inport  Port=2
  "n " : Inport  Port=3
  Constant : Constant  Value=0
  Core controller: Torque,Power and Combined Torque/Power : MATLAB Function  TreatAsAtomicUnit=on
  Integrator : Integrator  ExternalReset=either
  Ki : Gain  Gain=Kp/0.05
  Kp : Gain  Gain=Kp
  Sum : Sum  Inputs=+|-
  Sum1 : Sum  Inputs=|++
  Q_cn : Outport
  Qcq : Outport  Port=2
  Qcp : Outport  Port=3
  Qcc : Outport  Port=4
  wires:
  [Kq2r] -> Core controller: Torque,Power and Combined Torque/Power/12(K_q0r)
  [Kt2r] -> Core controller: Torque,Power and Combined Torque/Power/11(K_t0r)
  [eps_c] -> Core controller: Torque,Power and Combined Torque/Power/10(eps_c)
  Core controller: Torque,Power and Combined Torque/Power/1(Qcq) -> Qcq/1
  Core controller: Torque,Power and Combined Torque/Power/2(Qcp) -> Qcp/1
  "Tr "/1 -> Core controller: Torque,Power and Combined Torque/Power/8(Tr)
  "n "/1 -> Sum/2, Core controller: Torque,Power and Combined Torque/Power/4(n)
  [Rho] -> Core controller: Torque,Power and Combined Torque/Power/9(rho)
  [Kq2f] -> Core controller: Torque,Power and Combined Torque/Power/6(K_q0)
  [D] -> Core controller: Torque,Power and Combined Torque/Power/7(D)
  [Kt2f] -> Core controller: Torque,Power and Combined Torque/Power/5(K_t0)
  Core controller: Torque,Power and Combined Torque/Power/3(Qcc) -> Qcc/1
  [r_cc] -> Core controller: Torque,Power and Combined Torque/Power/3(r_cc)
  [p_cc] -> Core controller: Torque,Power and Combined Torque/Power/2(p_cc)
  [k_cc] -> Core controller: Torque,Power and Combined Torque/Power/1(k_cc)
  Constant/1 -> Integrator/2
  Sum1/1 -> Q_cn/1
  Sum/1 -> Kp/1, Ki/1
  Integrator/1 -> Sum1/2
  Kp/1 -> Sum1/1
  Ki/1 -> Integrator/1
  n_r/1 -> Sum/1

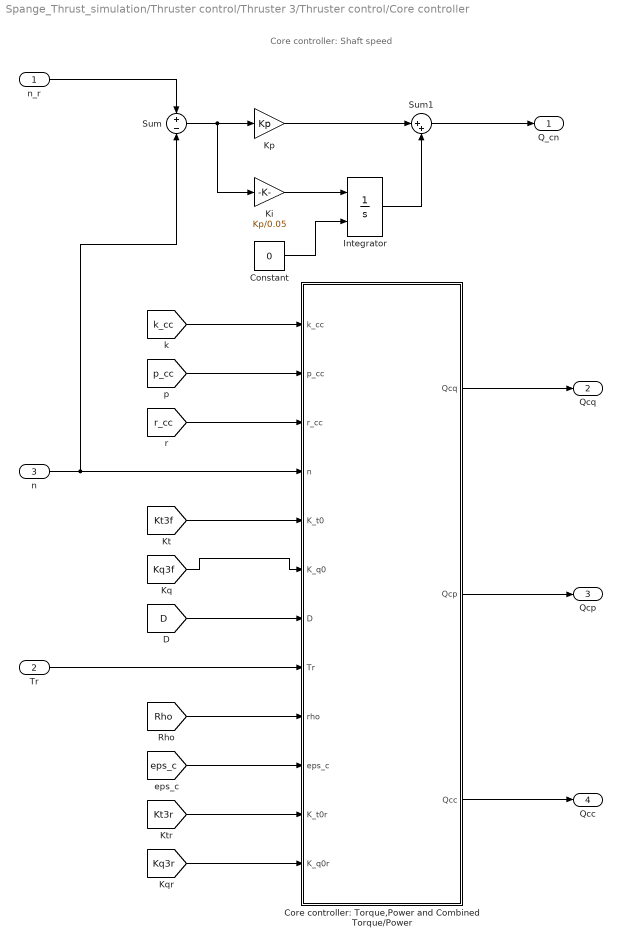
== system Spange_Thrust_simulation/Thruster control/Thruster 3/Thruster control/Core controller ==
  note: Core controller: Shaft speed
  n_r : Inport
  "Tr " : Inport  Port=2
  "n " : Inport  Port=3
  Constant : Constant  Value=0
  Core controller: Torque,Power and Combined Torque/Power : MATLAB Function  TreatAsAtomicUnit=on
  Integrator : Integrator  ExternalReset=either
  Ki : Gain  Gain=Kp/0.05
  Kp : Gain  Gain=Kp
  Sum : Sum  Inputs=+|-
  Sum1 : Sum  Inputs=|++
  Q_cn : Outport
  Qcq : Outport  Port=2
  Qcp : Outport  Port=3
  Qcc : Outport  Port=4
  wires:
  [Kq3r] -> Core controller: Torque,Power and Combined Torque/Power/12(K_q0r)
  [Kt3r] -> Core controller: Torque,Power and Combined Torque/Power/11(K_t0r)
  [eps_c] -> Core controller: Torque,Power and Combined Torque/Power/10(eps_c)
  Core controller: Torque,Power and Combined Torque/Power/1(Qcq) -> Qcq/1
  Core controller: Torque,Power and Combined Torque/Power/2(Qcp) -> Qcp/1
  "Tr "/1 -> Core controller: Torque,Power and Combined Torque/Power/8(Tr)
  "n "/1 -> Core controller: Torque,Power and Combined Torque/Power/4(n), Sum/2
  [Rho] -> Core controller: Torque,Power and Combined Torque/Power/9(rho)
  [Kq3f] -> Core controller: Torque,Power and Combined Torque/Power/6(K_q0)
  [D] -> Core controller: Torque,Power and Combined Torque/Power/7(D)
  [Kt3f] -> Core controller: Torque,Power and Combined Torque/Power/5(K_t0)
  Core controller: Torque,Power and Combined Torque/Power/3(Qcc) -> Qcc/1
  [r_cc] -> Core controller: Torque,Power and Combined Torque/Power/3(r_cc)
  [p_cc] -> Core controller: Torque,Power and Combined Torque/Power/2(p_cc)
  [k_cc] -> Core controller: Torque,Power and Combined Torque/Power/1(k_cc)
  Constant/1 -> Integrator/2
  Sum1/1 -> Q_cn/1
  Sum/1 -> Kp/1, Ki/1
  Integrator/1 -> Sum1/2
  Kp/1 -> Sum1/1
  Ki/1 -> Integrator/1
  n_r/1 -> Sum/1

== matlab function Spange_Thrust_simulation/T(F,alpha)/MATLAB Function ==
  data: thrust_actual input; actual_tau output; alpha_actual input; PosX input; PosY input
function actual_tau   = fcn(thrust_actual,alpha_actual,PosX,PosY)
%#codegen

Alpha_surge =[cosd(alpha_actual(1)) cosd(alpha_actual(2)) cosd(alpha_actual(3))];  
Alpha_sway = [sind(alpha_actual(1)) sind(alpha_actual(2)) sind(alpha_actual(3))];
Alpha_yaw = [sind(alpha_actual(1))*PosX(1)-cosd(alpha_actual(1))*PosY(1) sind(alpha_actual(2))*PosX(2)-cosd(alpha_actual(2))*PosY(2) ...
             sind(alpha_actual(3))*PosX(3)-cosd(alpha_actual(3))*PosY(3)];

actual_tau = [Alpha_surge;Alpha_sway;Alpha_yaw]*thrust_actual;

== matlab function Spange_Thrust_simulation/Thrus & angle aloc/For Each Subsystem/Ensures fastest way is chosen ==
  data: desired input; psi_D output; actual input
function psi_D   = OptimalAngle(desired,actual)
%#codegen
psi_D = desired-actual;
if abs(psi_D) >= 360
    psi_D = rem(psi_D,360);
end

if abs(psi_D) >= 180
    psi_D = psi_D - sign(psi_D)*360;
end

== matlab function Spange_Thrust_simulation/Thruster control/Thruster 1/Propeller Hydrodynamics/Actual Force and Torque ==
  data: Ta output; n input; Qa output; Kq input; Kt input; Ktr input; Kqr input; Rho input; D input; eps_c input; env input
function [Ta,Qa]= ActualForces(n,Kq,Kt,Ktr,Kqr,Rho,D,eps_c,env)
%#codegen
lambda_c = 0.5+0.5*tanh(eps_c*n/5); % Smooth switching between positive and negative thrust. 5 makes switch happen between -5 and 5
K_TC = Kt*lambda_c+(1-lambda_c)*Ktr;
K_QC = Kq*lambda_c+(1-lambda_c)*Kqr;

Ta = sign(n)*K_TC*Rho*(D^4)*n^2-env;
Qa = sign(n)*K_QC*Rho*(D^5)*n^2-env;

== matlab function Spange_Thrust_simulation/Thruster control/Thruster 1/Thruster control/Core controller/Core controller: Torque,Power and Combined Torque//Power ==
  data: Qcq output; Qcp output; k_cc input; p_cc input; r_cc input; n input; Qcc output; K_t0 input; K_q0 input; D input; Tr input; rho input; eps_c input; K_t0r input; K_q0r input
 function [Qcq,Qcp,Qcc]= CoreControl(k_cc,p_cc,r_cc,n,K_t0,K_q0,D,Tr,rho,eps_c,K_t0r,K_q0r)
%#codegen

lambda_c = 0.5+0.5*tanh(eps_c*n/5);
K_TC = K_t0*lambda_c+(1-lambda_c)*K_t0r;
K_QC = K_q0*lambda_c+(1-lambda_c)*K_q0r;
Qcq = (K_QC/K_TC)*D*Tr;
if n == 0
    Qcp = 0;
else
Qcp = sign(Tr)*K_QC*(abs(Tr)^(3/2))/(sqrt(rho)*D*K_TC^(3/2)*abs(n));
end
alpha_c = exp(-k_cc*abs(p_cc*n)^r_cc);

Qcc = alpha_c*Qcq + (1-alpha_c)*Qcp;

== matlab function Spange_Thrust_simulation/Thruster control/Thruster 1/Thruster control/MATLAB Function ==
  data: Td input; n_d output; K_t0 input; K_t0r input; rho input; D input; eps_c input; n_c input; n_r input; T_r output
function [n_d,T_r]  = ReferenceGenerator(Td,K_t0,K_t0r,rho,D,eps_c,n_c,n_r)
%#codegen


n_d = sign(Td)*sqrt((abs(Td))/(rho*D^4*K_t0));

lambda_c = 0.5+0.5*tanh(eps_c*n_r/n_c); % Smooth switching between positive and negative thrust.
K_TC = K_t0*lambda_c+(1-lambda_c)*K_t0r;

T_r = sign(n_r)*K_TC*rho*D^4*n_r^2;

== matlab function Spange_Thrust_simulation/Thrus & angle aloc/For Each Subsystem/MATLAB Function ==
  data: angle input; y output
function y = rad2pipi(angle)
% RAD2PIPI Converts an angle in rad to the interval (-pi pi]
%          Should be applied to all heading errors in a feedback control system
%          in order to avoid discontinuities.
%
% Author:     Roger Skjetne
% Date:       2003-09-05
% Revisions:  2004-09-02 Thor I. Fossen - replaced input argument x with angle
%             2005-01-05 Thor I. Fossen - ouput argument is set to y and not angle
%             2005-04-13 Roger Skjetne  - changed the function s in order
%                                         to account for correct mapping to
%                                         (-pi pi].
%
% ________________________________________________________________
%
% MSS GNC is a Matlab toolbox for guidance, navigation and control.
% The toolbox is part of the Marine Systems Simulator (MSS).
%
% Copyright (C) 2008 Thor I. Fossen and Tristan Perez
% 
% This program is free software: you can redistribute it and/or modify
% it under the terms of the GNU General Public License as published by
% the Free Software Foundation, either version 3 of the License, or
% (at your option) any later version.
% 
% This program is distributed in the hope that it will be useful, but
% WITHOUT ANY WARRANTY; without even the implied warranty of
% MERCHANTABILITY or FITNESS FOR A PARTICULAR PURPOSE.  See the 
% GNU General Public License for more details.
% 
% You should have received a copy of the GNU General Public License
% along with this program.  If not, see <http://www.gnu.org/licenses/>.
% 
% E-mail: contact@marinecontrol.org
% URL:    <http://www.marinecontrol.org>


% convert angle in rad to the interval <-pi pi> 
r = rem(angle+sign(angle)*pi,2*pi);
s = sign(sign(angle) + 2*(sign(abs(rem(angle+pi,2*pi)/(2*pi)))-1));
% s = sign(angle);

y = r - s*pi;

== matlab function Spange_Thrust_simulation/Thruster control/Thruster 1/Thruster control/Supervisor ==
  data: control input; input input; n input; u output
function u = fcn(control,input,n)
u = 1;
if control == 1
if input == 1
    u = 1;
elseif input == 2
    u = 2;
elseif input == 3 && n > 0.01 || input == 3 && n < -0.01
    u = 3;
elseif input == 4 || input == 3 && n < 0.01 || input == 3 && n > -0.01
    u = 4;
else 
    u = 5;
end
end

if control == 2
if input == 1
    u = 1;
elseif input == 2
    u = 2;
elseif input == 3 && n > 0.01 || input == 3 && n < -0.01
    u = 3;
elseif input == 4 || input == 3 && n < 0.01 || input == 3 && n > -0.01
    u = 4;
else 
    u = 5;
end
end

if control == 3
if input == 1
    u = 1;
elseif input == 2
    u = 2;
elseif input == 3 && n > 0.01 || input == 3 && n < -0.01
    u = 3;
elseif input == 4 || input == 3 && n < 0.01 || input == 3 && n > -0.01
    u = 4;
else 
    u = 5;
end
end

if control == 4
if input == 1
    u = 1;
elseif input == 2
    u = 2;
elseif input == 3 && n > 0.01 || input == 3 && n < -0.01
    u = 3;
elseif input == 4 || input == 3 && n < 0.01 || input == 3 && n > -0.01
    u = 4;
else 
    u = 5;
end
end

if control == 5
if input == 1
    u = 1;
elseif input == 2
    u = 2;
elseif input == 3 && n > 0.01 || input == 3 && n < -0.01
    u = 3;
elseif input == 4 || input == 3 && n < 0.01 || input == 3 && n > -0.01
    u = 4;
else 
    u = 5;
end
end

== matlab function Spange_Thrust_simulation/Thruster control/Thruster 2/Propeller Hydrodynamics/Actual Force and Torque ==
  data: Ta output; n input; Qa output; Kq input; Kt input; Ktr input; Kqr input; Rho input; D input; eps_c input; env input
function [Ta,Qa]= ActualForces(n,Kq,Kt,Ktr,Kqr,Rho,D,eps_c,env)
%#codegen
lambda_c = 0.5+0.5*tanh(eps_c*n/5); % Smooth switching between positive and negative thrust. 5 makes switch happen between -5 and 5
K_TC = Kt*lambda_c+(1-lambda_c)*Ktr;
K_QC = Kq*lambda_c+(1-lambda_c)*Kqr;

Ta = sign(n)*K_TC*Rho*(D^4)*n^2-env;
Qa = sign(n)*K_QC*Rho*(D^5)*n^2-env;

== matlab function Spange_Thrust_simulation/Thruster control/Thruster 2/Thruster control/Core controller/Core controller: Torque,Power and Combined Torque//Power ==
  data: Qcq output; Qcp output; k_cc input; p_cc input; r_cc input; n input; Qcc output; K_t0 input; K_q0 input; D input; Tr input; rho input; eps_c input; K_t0r input; K_q0r input
function [Qcq,Qcp,Qcc]= CoreControl(k_cc,p_cc,r_cc,n,K_t0,K_q0,D,Tr,rho,eps_c,K_t0r,K_q0r)
%#codegen

lambda_c = 0.5+0.5*tanh(eps_c*n/5);
K_TC = K_t0*lambda_c+(1-lambda_c)*K_t0r;
K_QC = K_q0*lambda_c+(1-lambda_c)*K_q0r;
Qcq = (K_QC/K_TC)*D*Tr;
if n == 0
    Qcp = 0;
else
Qcp = sign(Tr)*K_QC*(abs(Tr)^(3/2))/(sqrt(rho)*D*K_TC^(3/2)*abs(n));
end
alpha_c = exp(-k_cc*abs(p_cc*n)^r_cc);

Qcc = alpha_c*Qcq + (1-alpha_c)*Qcp;

== matlab function Spange_Thrust_simulation/Thruster control/Thruster 2/Thruster control/MATLAB Function ==
  data: Td input; n_d output; K_t0 input; K_t0r input; rho input; D input; eps_c input; n_c input; n_r input; T_r output
function [n_d,T_r]  = ReferenceGenerator(Td,K_t0,K_t0r,rho,D,eps_c,n_c,n_r)
%#codegen


n_d = sign(Td)*sqrt((abs(Td))/(rho*D^4*K_t0));

lambda_c = 0.5+0.5*tanh(eps_c*n_r/n_c); % Smooth switching between positive and negative thrust. 
K_TC = K_t0*lambda_c+(1-lambda_c)*K_t0r;

T_r = sign(n_r)*K_TC*rho*D^4*n_r^2;

== matlab function Spange_Thrust_simulation/Thruster control/Thruster 2/Thruster control/Supervisor ==
  data: control input; input input; n input; u output
function u = fcn(control,input,n)
u = 1;
if control == 1
if input == 1
    u = 1;
elseif input == 2
    u = 2;
elseif input == 3 && n > 0.01 || input == 3 && n < -0.01
    u = 3;
elseif input == 4 || input == 3 && n < 0.01 || input == 3 && n > -0.01
    u = 4;
else 
    u = 5;
end
end

if control == 2
if input == 1
    u = 1;
elseif input == 2
    u = 2;
elseif input == 3 && n > 0.01 || input == 3 && n < -0.01
    u = 3;
elseif input == 4 || input == 3 && n < 0.01 || input == 3 && n > -0.01
    u = 4;
else 
    u = 5;
end
end

if control == 3
if input == 1
    u = 1;
elseif input == 2
    u = 2;
elseif input == 3 && n > 0.01 || input == 3 && n < -0.01
    u = 3;
elseif input == 4 || input == 3 && n < 0.01 || input == 3 && n > -0.01
    u = 4;
else 
    u = 5;
end
end

if control == 4
if input == 1
    u = 1;
elseif input == 2
    u = 2;
elseif input == 3 && n > 0.01 || input == 3 && n < -0.01
    u = 3;
elseif input == 4 || input == 3 && n < 0.01 || input == 3 && n > -0.01
    u = 4;
else 
    u = 5;
end
end

if control == 5
if input == 1
    u = 1;
elseif input == 2
    u = 2;
elseif input == 3 && n > 0.01 || input == 3 && n < -0.01
    u = 3;
elseif input == 4 || input == 3 && n < 0.01 || input == 3 && n > -0.01
    u = 4;
else 
    u = 5;
end
end

== matlab function Spange_Thrust_simulation/Thruster control/Thruster 3/Propeller Hydrodynamics/Actual Force and Torque ==
  data: Ta output; n input; Qa output; Kq input; Kt input; Ktr input; Kqr input; Rho input; D input; eps_c input; env input
function [Ta,Qa]= ActualForces(n,Kq,Kt,Ktr,Kqr,Rho,D,eps_c,env)
%#codegen
lambda_c = 0.5+0.5*tanh(eps_c*n/5); % Smooth switching between positive and negative thrust. 5 makes switch happen between -5 and 5
K_TC = Kt*lambda_c+(1-lambda_c)*Ktr;
K_QC = Kq*lambda_c+(1-lambda_c)*Kqr;

Ta = sign(n)*K_TC*Rho*(D^4)*n^2-env;
Qa = sign(n)*K_QC*Rho*(D^5)*n^2-env;

== matlab function Spange_Thrust_simulation/Thruster control/Thruster 3/Thruster control/Core controller/Core controller: Torque,Power and Combined Torque//Power ==
  data: Qcq output; Qcp output; k_cc input; p_cc input; r_cc input; n input; Qcc output; K_t0 input; K_q0 input; D input; Tr input; rho input; eps_c input; K_t0r input; K_q0r input
function [Qcq,Qcp,Qcc]= CoreControl(k_cc,p_cc,r_cc,n,K_t0,K_q0,D,Tr,rho,eps_c,K_t0r,K_q0r)
%#codegen

lambda_c = 0.5+0.5*tanh(eps_c*n/5);
K_TC = K_t0*lambda_c+(1-lambda_c)*K_t0r;
K_QC = K_q0*lambda_c+(1-lambda_c)*K_q0r;
Qcq = (K_QC/K_TC)*D*Tr;
if n == 0
    Qcp = 0;
else
Qcp = sign(Tr)*K_QC*(abs(Tr)^(3/2))/(sqrt(rho)*D*K_TC^(3/2)*abs(n));
end
alpha_c = exp(-k_cc*abs(p_cc*n)^r_cc);

Qcc = alpha_c*Qcq + (1-alpha_c)*Qcp;

== matlab function Spange_Thrust_simulation/Thruster control/Thruster 3/Thruster control/MATLAB Function ==
  data: Td input; n_d output; K_t0 input; K_t0r input; rho input; D input; eps_c input; n_c input; n_r input; T_r output
function [n_d,T_r]  = ReferenceGenerator(Td,K_t0,K_t0r,rho,D,eps_c,n_c,n_r)
%#codegen


n_d = sign(Td)*sqrt((abs(Td))/(rho*D^4*K_t0));

lambda_c = 0.5+0.5*tanh(eps_c*n_r/n_c); % Smooth switching between positive and negative thrust.
K_TC = K_t0*lambda_c+(1-lambda_c)*K_t0r;

T_r = sign(n_r)*K_TC*rho*D^4*n_r^2;

== matlab function Spange_Thrust_simulation/Thruster control/Thruster 3/Thruster control/Supervisor ==
  data: control input; input input; n input; u output
function u = fcn(control,input,n)
u = 1;
if control == 1
if input == 1
    u = 1;
elseif input == 2
    u = 2;
elseif input == 3 && n > 0.01 || input == 3 && n < -0.01
    u = 3;
elseif input == 4 || input == 3 && n < 0.01 || input == 3 && n > -0.01
    u = 4;
else 
    u = 5;
end
end

if control == 2
if input == 1
    u = 1;
elseif input == 2
    u = 2;
elseif input == 3 && n > 0.01 || input == 3 && n < -0.01
    u = 3;
elseif input == 4 || input == 3 && n < 0.01 || input == 3 && n > -0.01
    u = 4;
else 
    u = 5;
end
end

if control == 3
if input == 1
    u = 1;
elseif input == 2
    u = 2;
elseif input == 3 && n > 0.01 || input == 3 && n < -0.01
    u = 3;
elseif input == 4 || input == 3 && n < 0.01 || input == 3 && n > -0.01
    u = 4;
else 
    u = 5;
end
end

if control == 4
if input == 1
    u = 1;
elseif input == 2
    u = 2;
elseif input == 3 && n > 0.01 || input == 3 && n < -0.01
    u = 3;
elseif input == 4 || input == 3 && n < 0.01 || input == 3 && n > -0.01
    u = 4;
else 
    u = 5;
end
end

if control == 5
if input == 1
    u = 1;
elseif input == 2
    u = 2;
elseif input == 3 && n > 0.01 || input == 3 && n < -0.01
    u = 3;
elseif input == 4 || input == 3 && n < 0.01 || input == 3 && n > -0.01
    u = 4;
else 
    u = 5;
end
end
